simulink model "test01b"  (Simulink 4.00)
settings: Solver=FixedStepDiscrete  StartTime=0.0  StopTime=120  FixedStep=1/4000  RelTol=1e-3
settings Model: Creator=root  LastModifiedBy=root  SimulationMode=external  RTWSystemTargetFile=wintarget.tlc  RTWOptions="-aEnforceIntegerDowncast=1 -aExtMode=1 -aFoldNonRolledExpr=1 -aForceParamTrailComments=0 -aGenerateComments=1 -aIgnoreCustomStorageClasses=1 -aIncHierarchyInIds=0 -aInlineInvariantSignals=0 -aInlineParameters=0 -aLocalBlockOutputs=1 -aLogVarNameModifier=\"rt_\" -aRTWVerbose=1 -aRollThreshold=5 -aShowEliminatedStatements=1"  RTWTemplateMakefile=wt_default_tmf  ExtModeAutoUpdateStatusClock=off

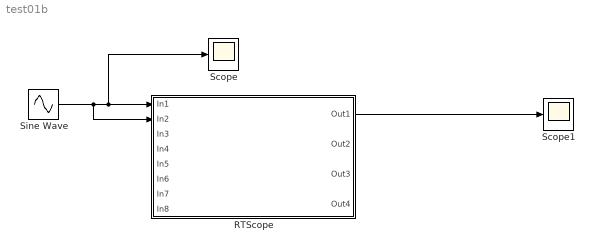
== system test01b ==
  RTScope : Subsystem
      settings: OpenFcn=rtscope  RTWFcnNameOpts=Auto  RTWFileNameOpts=Auto
      mask Type: RTScope
      mask Display: image(imread('rtscope2.jpg'))
  Scope : Scope
      settings: TimeRange=1  YMin=-5  YMax=5  SaveToWorkspace=off  SaveName=ScopeData  LimitDataPoints=on  MaxDataPoints=5000
  Scope1 : Scope
      settings: TimeRange=1  YMin=-1  YMax=1  SaveToWorkspace=off  LimitDataPoints=on  MaxDataPoints=5000
  Sine Wave : Sin  SineType=Time-based  Amplitude=3  Bias=0  Frequency=2*pi*10  Phase=0  Samples=10  SampleTime=0  Offset=0
  wires:
  Sine Wave/1 -> Scope/1, RTScope/1(In1), RTScope/2(In2)
  RTScope/1(Out1) -> Scope1/1

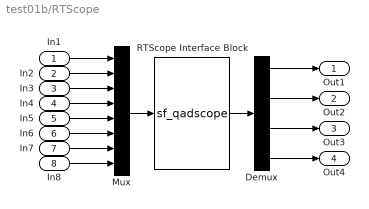
== system test01b/RTScope ==
  In1 : Inport  Port=1  LatchInput=off
  In2 : Inport  Port=2  LatchInput=off
  In3 : Inport  Port=3  LatchInput=off
  In4 : Inport  Port=4  LatchInput=off
  In5 : Inport  Port=5  LatchInput=off
  In6 : Inport  Port=6  LatchInput=off
  In7 : Inport  Port=7  LatchInput=off
  In8 : Inport  Port=8  LatchInput=off
  Demux : Demux  Outputs=4  BusSelectionMode=off
  Mux : Mux  Inputs=8
  RTScope Interface Block : S-Function  FunctionName=sf_qadscope  Parameters=4000  PortCounts=[]  SFunctionModules=''
      settings: OpenFcn=rtscope
  Out1 : Outport  Port=1
  Out2 : Outport  Port=2
  Out3 : Outport  Port=3
  Out4 : Outport  Port=4
  wires:
  Mux/1 -> RTScope Interface Block/1
  RTScope Interface Block/1 -> Demux/1
  Demux/1 -> Out1/1
  Demux/2 -> Out2/1
  Demux/3 -> Out3/1
  Demux/4 -> Out4/1
  In1/1 -> Mux/1
  In2/1 -> Mux/2
  In3/1 -> Mux/3
  In4/1 -> Mux/4
  In5/1 -> Mux/5
  In6/1 -> Mux/6
  In7/1 -> Mux/7
  In8/1 -> Mux/8
